simulink model "pvinverter_pmodel"  (R2014a)
settings: Solver=FixedStepDiscrete  StartTime=0.0  StopTime=0.2  FixedStep=Ts  MaxStep=1e-3  RelTol=1e-4
PreLoadFcn:
  | PVArrayIsc = 5;
  | PVArrayVoc = 21.6;
  | PVArrayRs = 0.036;
  | Tcircuit = 27.15;
  | Toffset = -2;
  | TIPH1 = 0.001;
  | TXIS1 = 3;
  | TRS1 = 0;
  | Ts = 1e-6;
  | load('InvBusObject');
  | load('PVBusObject');
InitFcn:
  | Ts = 1e-6;
StartFcn:
  | tic;
StopFcn:
  | toc;
libraries: powerlib x13, powerlib_meascontrol x2
settings Model: Creator=cosorio  LastModifiedBy=cosorio
settings DataIOCC: LimitDataPoints=off  SignalLoggingSaveFormat=ModelDataLogs  SaveOutput=off  SignalLogging=off  SaveTime=off
settings OptimizationCC: InlineParams=on  ExpressionDepthLimit=2147483647
settings DebuggingCC: UnderspecifiedInitializationDetection=Classic  SolverPrmCheckMsg=none  FcnCallInpInsideContextMsg=UseLocalSettings  StateNameClashWarn=warning
settings GRTTargetCC: CombineOutputUpdateFcns=off  GRTInterface=on

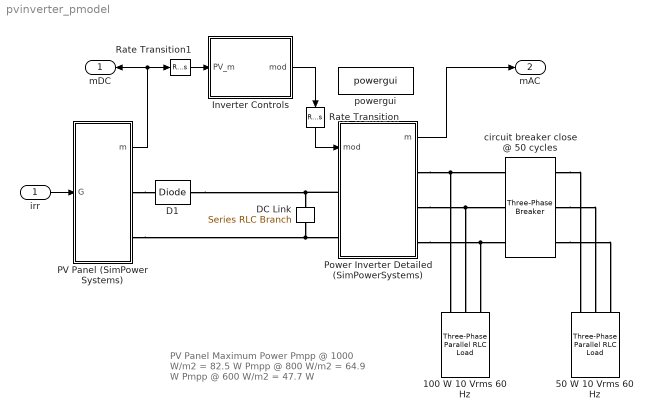
== system pvinverter_pmodel ==
  note: PV Panel Maximum Power
      | Pmpp @ 1000 W/m2 = 82.5 W
      | Pmpp @ 800 W/m2 = 64.9 W
      | Pmpp @ 600 W/m2 = 47.7 W
  irr : Inport  OutDataTypeStr=double  PortDimensions=1  SampleTime=Ts
  100 W 10 Vrms 60 Hz : powerlib/Elements/Three-Phase Parallel RLC Load  LConnTagsString=A|B|C  Configuration=Y (grounded)  NominalVoltage=10  NominalFrequency=60  ActivePower=100  InductivePower=0  CapacitivePower=0  Measurements=None  LoadType=constant Z
  50 W 10 Vrms 60 Hz : powerlib/Elements/Three-Phase Parallel RLC Load  LConnTagsString=A|B|C  Configuration=Y (grounded)  NominalVoltage=10  NominalFrequency=60  ActivePower=50  InductivePower=0  CapacitivePower=0  Measurements=None  LoadType=constant Z
  D1 : powerlib/Power Electronics/Diode  Ron=0.001  Lon=0  Vf=0.8  IC=0  UseSnubber=off  Rs=500  Cs=250e-9  Measurements=off
  DC Link : powerlib/Elements/Series RLC Branch  LConnTagsString=__new0  RConnTagsString=__new0  BranchType=C  Resistance=1  Inductance=1e-3  SetiL0=off  InitialCurrent=0  Capacitance=480e-6  Setx0=on  InitialVoltage=18  Measurements=None
  Inverter Controls : Subsystem  TreatAsAtomicUnit=on  SystemSampleTime=1e-4
  PV Panel (SimPowerSystems) : Subsystem
  Power Inverter Detailed (SimPowerSystems) : Subsystem
  Rate Transition : RateTransition
  Rate Transition1 : RateTransition
  circuit breaker close @ 50 cycles : powerlib/Elements/Three-Phase Breaker  InitialState=open  SwitchA=on  SwitchB=on  SwitchC=on  SwitchTimes=[50/60]  External=off  BreakerResistance=0.001  SnubberResistance=1e6  SnubberCapacitance=inf  Measurements=None
  powergui : powerlib/powergui  Priority=1  SimulationMode=Discrete  SolverType=Tustin  SampleTime=Ts  frequency=60  SPID=off  DisableSnubberDevices=off  DisableRonSwitches=off  DisableVfSwitches=off  SwTol=0  Interpol=off  DisplayEquations=off  Ts=0  methode=off  frequencyindice=0  Pbase=100e6  ErrMax=1e-4  Iterations=50  UnitsV=kV  UnitsW=MW  FunctionMessages=off  echomessages=off  HookPort=off  EnableUseOfTLC=on  x0status=blocks  RestoreLinks=warning  ResistiveCurrentMeasurement=off  Frange=[0:2:500]  Ylog=off  Xlog=on  ShowGrid=off  save=off  variable=ZData  structure=0  ZoomFFT=on  StartTime=0.0  cycles=1  DisplayStyle=1  fundamental=60  FreqAxis=off  MaxFrequency=1000  frequencyindicesteady=1  RmsSteady=1  display=off
  mDC : Outport  OutDataTypeStr=Bus: PVPanelMeasurements  SampleTime=Ts
  mAC : Outport  Port=2  OutDataTypeStr=Bus: InverterMeasurements  SampleTime=Ts
  wires:
  Inverter Controls/1(mod) -> Rate Transition/1
  Power Inverter Detailed (SimPowerSystems)/1(m) -> mAC/1
  PV Panel (SimPowerSystems)/1(m) -> mDC/1, Rate Transition1/1
  irr/1 -> PV Panel (SimPowerSystems)/1(G)
  Rate Transition/1 -> Power Inverter Detailed (SimPowerSystems)/1(mod)
  Rate Transition1/1 -> Inverter Controls/1(PV_m)
  connections:
  Power Inverter Detailed (SimPowerSystems)/RConn2 -- circuit breaker close @ 50 cycles/LConn2 -- 100 W 10 Vrms 60 Hz/LConn2
  Power Inverter Detailed (SimPowerSystems)/RConn1 -- circuit breaker close @ 50 cycles/LConn1 -- 100 W 10 Vrms 60 Hz/LConn1
  Power Inverter Detailed (SimPowerSystems)/RConn3 -- circuit breaker close @ 50 cycles/LConn3 -- 100 W 10 Vrms 60 Hz/LConn3
  DC Link/RConn1 -- Power Inverter Detailed (SimPowerSystems)/LConn2 -- PV Panel (SimPowerSystems)/RConn2
  Power Inverter Detailed (SimPowerSystems)/LConn1 -- DC Link/LConn1 -- D1/RConn1
  circuit breaker close @ 50 cycles/RConn1 -- 50 W 10 Vrms 60 Hz/LConn1
  circuit breaker close @ 50 cycles/RConn2 -- 50 W 10 Vrms 60 Hz/LConn2
  circuit breaker close @ 50 cycles/RConn3 -- 50 W 10 Vrms 60 Hz/LConn3
  PV Panel (SimPowerSystems)/RConn1 -- D1/LConn1

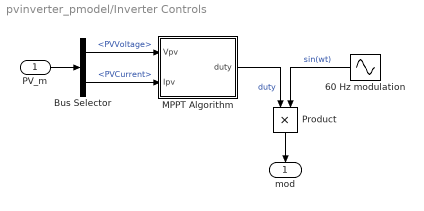
== system pvinverter_pmodel/Inverter Controls ==
  PV_m : Inport  OutDataTypeStr=Bus: PVPanelMeasurements  SampleTime=1e-4
  60 Hz modulation : Sin  Frequency=2*pi*60  Phase=[0, 120*pi/180, -120*pi/180]  SampleTime=1e-4
  Bus Selector : BusSelector  OutputSignals=PVVoltage,PVCurrent
  MPPT Algorithm : Subsystem
  Product : Product  RndMeth=Zero
  mod : Outport  PortDimensions=3  SampleTime=1e-4
  wires:
  MPPT Algorithm/1(duty) -> Product/1  "duty"
  Bus Selector/2 -> MPPT Algorithm/2(Ipv)  "<PVCurrent>"
  Bus Selector/1 -> MPPT Algorithm/1(Vpv)  "<PVVoltage>"
  Product/1 -> mod/1
  PV_m/1 -> Bus Selector/1
  60 Hz modulation/1 -> Product/2  "sin(wt)"

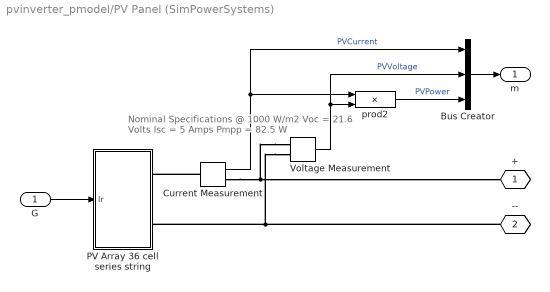
== system pvinverter_pmodel/PV Panel (SimPowerSystems) ==
  note: Nominal Specifications @ 1000 W/m2
      | Voc = 21.6 Volts
      | Isc = 5 Amps
      | Pmpp = 82.5 W
  G : Inport  OutDataTypeStr=double  PortDimensions=1  SampleTime=Ts
  Bus Creator : BusCreator  Inputs=3
  Current Measurement : powerlib/Measurements/Current Measurement  PhasorSimulation=off  OutputType=Complex  PSBequivalent=0
  PV Array 36 cell series string : Subsystem  mask(Solar Cell){Isc=5, Voc=0.6*36, Ir0=1000, N=1.5*36, Rs=0.001*36, Rp=1000*36, tau=Ts}
      mask prompts: Isc "Short-circuit current, Isc (A):"; Voc "Open-circuit voltage, Voc (V):"; Ir0 "Irradiance used for measurements, Ir0 (W/m2):"; N "Quality factor, N:"; Rs "Series resistance, Rs (ohms):"; Rp "Parallel resistance, Rp (ohms):"; tau "Time constant (sec):"
      mask help:
      | Simulink implementation of an idividual solar cell. The cell is modelled as a parallel combination of a current source, an exponential diode and an internal resistance Rp, connected in series with a resistance Rs.
      | The cell output current is given by:
      |
      | Ipv = Iph - Is * (exp((V + I*Rs)/(N*Vt)) - 1) - (V + I*Rs)/Rp
      |
      | Where Iph is the solar generated current, Is is the diode saturation current, Vt is the thermal voltage, N is the diode quality factor (emission coefficient).
      |
      | A first order transfer function is used to break the algebraic loop. The time constant of this transfer function should be adjusted such that it will not significantly affect your model dynamics.
      mask init:
      | %% Cell thermal voltage calculation
      | T = 25 + 273;   % Device operating temperature (oC)
      | k = 1.3806e-23; % Boltzman constant (J/oK)
      | q = 1.602e-19;  % Elementary charge on an electron (oC)
      | Vt = k*T/q;     % Thermal voltage
      | 
      | %% Diode saturation current calculation
      | Is = Isc/(exp(Voc/(N*Vt))-1);
  Voltage Measurement : powerlib/Measurements/Voltage Measurement  PhasorSimulation=off  OutputType=Complex  PSBequivalent=0
  prod2 : Product  Inputs=**
  + : PMIOPort  Tag=PMCPort  Port=1  Side=Right
  -- : PMIOPort  Tag=PMCPort  Port=2  Side=Right
  m : Outport  OutDataTypeStr=Bus: PVPanelMeasurements  SampleTime=Ts
  wires:
  Current Measurement/1 -> Bus Creator/1, prod2/1  "PVCurrent"
  Voltage Measurement/1 -> Bus Creator/2, prod2/2  "PVVoltage"
  Bus Creator/1 -> m/1
  G/1 -> PV Array 36 cell series string/1(Ir)
  prod2/1 -> Bus Creator/3  "PVPower"
  connections:
  Current Measurement/LConn1 -- PV Array 36 cell series string/RConn1
  Voltage Measurement/LConn1 -- +/RConn1 -- Current Measurement/RConn1
  Voltage Measurement/LConn2 -- PV Array 36 cell series string/RConn2 -- --/RConn1

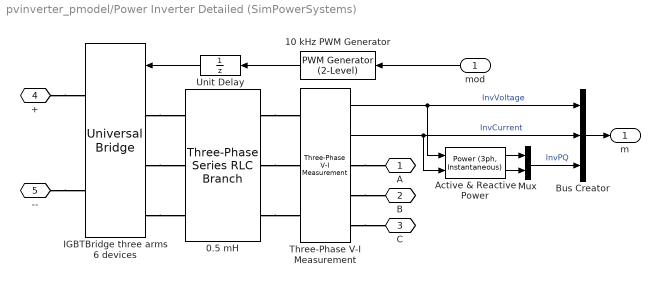
== system pvinverter_pmodel/Power Inverter Detailed (SimPowerSystems) ==
  mod : Inport  OutDataTypeStr=double  PortDimensions=3  SampleTime=Ts
  0.5 mH : powerlib/Elements/Three-Phase Series RLC Branch  LConnTagsString=A|B|C  RConnTagsString=A|B|C  BranchType=L  Resistance=1.0  Inductance=500e-6  Capacitance=1.0  Measurements=None
  10 kHz PWM Generator : powerlib_meascontrol/Pulse & Signal Generators/PWM Generator (2-Level)  ModulatorType=Three-phase bridge (6 pulses)  ModulatorMode=Unsynchronized  nF=27  Fc=1e4  ModulatingSignals=off  m=0.8  Freq=60  Phase=0  Ts=Ts
  Active & Reactive Power : powerlib_meascontrol/Measurements/Power (3ph, Instantaneous)
  Bus Creator : BusCreator  Inputs=3
  IGBTBridge three arms 6 devices : powerlib/Power Electronics/Universal Bridge  Arms=3  SnubberResistance=1e5  SnubberCapacitance=inf  Device=IGBT / Diodes  Ron=1e-3  Lon=0  ForwardVoltages="[  0  0  ]"  ForwardVoltage=0  GTOparameters=[ 10e-6 , 20e-6 ]  IGBTparameters=[ 1e-6 , 2e-6 ]  Measurements=None  Measurements_2=None  converterType=Rectifier
  Mux : Mux  Inputs=2
  Three-Phase V-I Measurement : powerlib/Measurements/Three-Phase V-I Measurement  VoltageMeasurement=phase-to-ground  SetLabelV=off  LabelV=Vabc  Vpu=off  VpuLL=off  CurrentMeasurement=yes  SetLabelI=off  LabelI=Iabc  Ipu=off  Pbase=100e6  Vbase=500e3  OutputType=Complex  PhasorSimulation=off  PSBequivalent=0
  Unit Delay : UnitDelay  SampleTime=Ts
  A : PMIOPort  Port=1  Side=Right
  B : PMIOPort  Port=2  Side=Right
  C : PMIOPort  Port=3  Side=Right
  + : PMIOPort  Port=4  Side=Left
  -- : PMIOPort  Port=5  Side=Left
  m : Outport  OutDataTypeStr=Bus: InverterMeasurements  SampleTime=Ts
  wires:
  10 kHz PWM Generator/1 -> Unit Delay/1
  Active & Reactive Power/1 -> Mux/1
  Active & Reactive Power/2 -> Mux/2
  Unit Delay/1 -> IGBTBridge three arms 6 devices/1
  mod/1 -> 10 kHz PWM Generator/1
  Bus Creator/1 -> m/1
  Three-Phase V-I Measurement/2 -> Active & Reactive Power/2, Bus Creator/2  "InvCurrent"
  Mux/1 -> Bus Creator/3  "InvPQ"
  Three-Phase V-I Measurement/1 -> Active & Reactive Power/1, Bus Creator/1  "InvVoltage"
  connections:
  --/RConn1 -- IGBTBridge three arms 6 devices/RConn2
  +/RConn1 -- IGBTBridge three arms 6 devices/RConn1
  Three-Phase V-I Measurement/RConn3 -- C/RConn1
  Three-Phase V-I Measurement/RConn2 -- B/RConn1
  Three-Phase V-I Measurement/RConn1 -- A/RConn1
  0.5 mH/RConn3 -- Three-Phase V-I Measurement/LConn3
  0.5 mH/RConn2 -- Three-Phase V-I Measurement/LConn2
  0.5 mH/RConn1 -- Three-Phase V-I Measurement/LConn1
  IGBTBridge three arms 6 devices/LConn3 -- 0.5 mH/LConn3
  IGBTBridge three arms 6 devices/LConn2 -- 0.5 mH/LConn2
  IGBTBridge three arms 6 devices/LConn1 -- 0.5 mH/LConn1

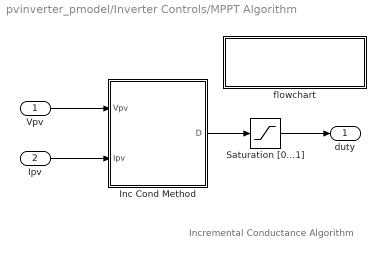
== system pvinverter_pmodel/Inverter Controls/MPPT Algorithm ==
  note: Incremental Conductance Algorithm
  Vpv : Inport  OutDataTypeStr=double  PortDimensions=1  SampleTime=[0.0001,0]
  Ipv : Inport  Port=2  OutDataTypeStr=double  PortDimensions=1  SampleTime=[0.0001,0]
  Inc Cond Method : Stateflow chart  TreatAsAtomicUnit=on
  Saturation [0...1] : Saturate  UpperLimit=1  LowerLimit=0
  flowchart : Subsystem
      settings: OpenFcn=winopen('INC.jpg');
      mask Display: disp('Algorithm\nFlowchart')
  duty : Outport  OutDataTypeStr=double  PortDimensions=1  SampleTime=[0.0001,0]
  wires:
  Saturation [0...1]/1 -> duty/1
  Ipv/1 -> Inc Cond Method/2(Ipv)
  Vpv/1 -> Inc Cond Method/1(Vpv)
  Inc Cond Method/1(D) -> Saturation [0...1]/1

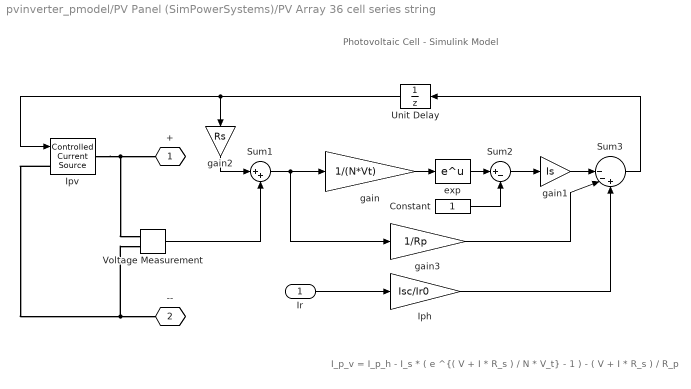
== system pvinverter_pmodel/PV Panel (SimPowerSystems)/PV Array 36 cell series string ==
  note: Photovoltaic Cell - Simulink Model
  note: I_p_v = I_p_h - I_s * ( e ^{( V + I * R_s ) / N * V_t} - 1 ) - ( V + I * R_s ) / R_p
  Ir : Inport
  Constant : Constant
  Iph : Gain  Gain=Isc/Ir0
  Ipv : powerlib/Electrical Sources/Controlled Current Source  Initialize=on  Source_Type=DC  Amplitude=0  Phase=0  Frequency=0  Measurements=None
  Sum1 : Sum  Inputs=|++
  Sum2 : Sum  Inputs=|+-
  Sum3 : Sum  Inputs=||--+
  Unit Delay : UnitDelay  InitialCondition=4.65  SampleTime=tau
  Voltage Measurement : powerlib/Measurements/Voltage Measurement  PhasorSimulation=off  OutputType=Complex  PSBequivalent=0
  exp : Math  SaturateOnIntegerOverflow=on
  gain : Gain  Gain=1/(N*Vt)
  gain1 : Gain  Gain=Is
  gain2 : Gain  Gain=Rs
  gain3 : Gain  Gain=1/Rp
  + : PMIOPort  Tag=PMCPort  Port=1  Side=Right
  -- : PMIOPort  Tag=PMCPort  Port=2  Side=Right
  wires:
  Iph/1 -> Sum3/3
  gain3/1 -> Sum3/2
  gain1/1 -> Sum3/1
  gain2/1 -> Sum1/1
  Unit Delay/1 -> Ipv/1, gain2/1
  Ir/1 -> Iph/1
  Voltage Measurement/1 -> Sum1/2
  Sum3/1 -> Unit Delay/1
  gain/1 -> exp/1
  Sum1/1 -> gain3/1, gain/1
  exp/1 -> Sum2/1
  Constant/1 -> Sum2/2
  Sum2/1 -> gain1/1
  connections:
  Ipv/LConn1 -- --/RConn1 -- Voltage Measurement/LConn2
  Ipv/RConn1 -- +/RConn1 -- Voltage Measurement/LConn1

== system pvinverter_pmodel/Inverter Controls/MPPT Algorithm/flowchart ==

== stateflow chart pvinverter_pmodel/Inverter Controls/MPPT Algorithm/Inc Cond Method ==
  settings: updateMethod=DISCRETE  sampleTime=1e-4
  state SAMPLEandCALCULATE
    entry:
    deltaV = Vpv - Vprev;
    deltaI = Ipv - Iprev;
    d = D;
  state INCREMENT_DUTY
    entry:
    d = d + deltad;
  state DECREMENT_DUTY
    entry:
    d = d - deltad;
  state RETURN
    entry:
    Vprev = Vpv; Iprev = Ipv;
    D = d;
  RETURN -> SAMPLEandCALCULATE
  (default) -> SAMPLEandCALCULATE
  SAMPLEandCALCULATE -> (junction 14) [order 1] : [deltaV > Vtol || deltaV < -Vtol]
  SAMPLEandCALCULATE -> (junction 15) [order 2]
  (junction 15) -> RETURN [order 3]
  (junction 15) -> INCREMENT_DUTY [order 1] : [deltaI < -Itol]
  (junction 14) -> RETURN [order 3]
  (junction 14) -> DECREMENT_DUTY [order 1] : [deltaI/deltaV > -Ipv/Vpv]
  (junction 14) -> INCREMENT_DUTY [order 2] : [deltaI/deltaV < -Ipv/Vpv]
  (junction 15) -> DECREMENT_DUTY [order 2] : [deltaI > Itol]
  INCREMENT_DUTY -> RETURN
  DECREMENT_DUTY -> RETURN
  data: Vpv input; Ipv input; D output double =0.8; Vprev local double =0; Iprev local double =0; Itol constant double =0.001; Vtol constant double =0.001; deltad constant double =0.0025; deltaV local double =0; deltaI local double =0; d local double =0
